simulink model "shock_absorb"  (R2020b)
settings: Solver=VariableStepAuto  StartTime=0.0  StopTime=100  RelTol=1e-3
model workspace (MAT data in the model file):
  b = Simulink.Parameter
  b.Value = 8
  b.DataType = 'auto'
  b.Dimensions = [1 1]
  k1 = Simulink.Parameter
  k1.Value = 5.71
  k1.DataType = 'auto'
  k1.Dimensions = [1 1]
  k2 = Simulink.Parameter
  k2.Value = 0.15
  k2.DataType = 'auto'
  k2.Dimensions = [1 1]
  m1 = Simulink.Parameter
  m1.Value = 330
  m1.DataType = 'auto'
  m1.Dimensions = [1 1]
  m2 = Simulink.Parameter
  m2.Value = 165
  m2.DataType = 'auto'
  m2.Dimensions = [1 1]
settings Model: Creator=shivanshu shukla  LastModifiedBy=shivanshu shukla

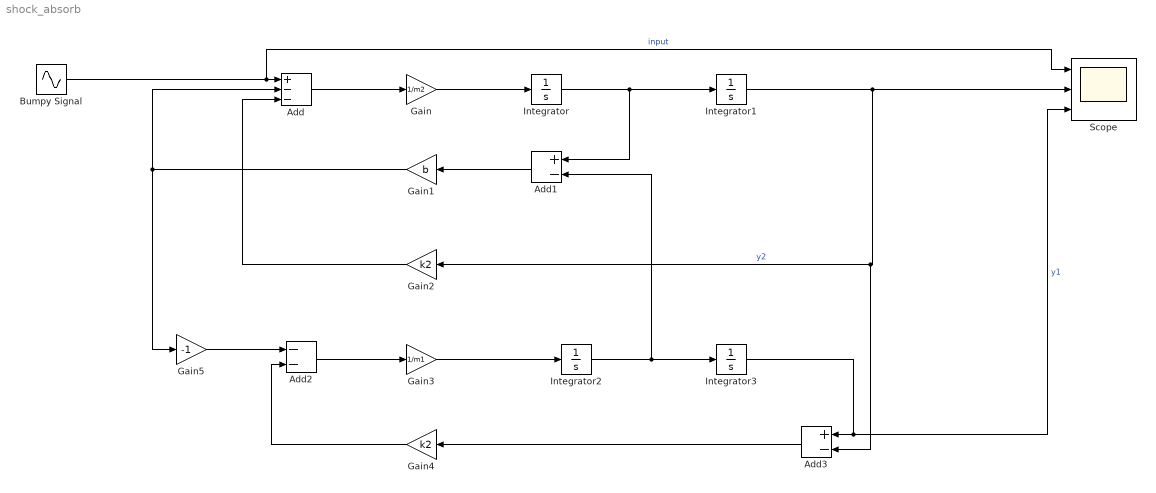
== system shock_absorb ==
  Add : Sum  Inputs=+--
  Add1 : Sum  Inputs=+-
  Add2 : Sum  Inputs=--
  Add3 : Sum  Inputs=+-
  Bumpy Signal : Sin  SampleTime=0
  Gain : Gain  Gain=1/m2
  Gain1 : Gain  Gain=b
  Gain2 : Gain  Gain=k2
  Gain3 : Gain  Gain=1/m1
  Gain4 : Gain  Gain=k2
  Gain5 : Gain  Gain=-1
  Integrator{,1..3} (4 alike) : Integrator
  Scope : Scope  NumInputPorts=3
  wires:
  Add/1 -> Gain/1
  Gain/1 -> Integrator/1
  Integrator/1 -> Add1/1, Integrator1/1
  Integrator1/1 -> Scope/2, Gain2/1, Add3/2  "y2"
  Gain1/1 -> Gain5/1, Add/2
  Add1/1 -> Gain1/1
  Gain2/1 -> Add/3
  Gain3/1 -> Integrator2/1
  Integrator2/1 -> Add1/2, Integrator3/1
  Gain5/1 -> Add2/1
  Add2/1 -> Gain3/1
  Integrator3/1 -> Scope/3, Add3/1  "y1"
  Add3/1 -> Gain4/1
  Gain4/1 -> Add2/2
  Bumpy Signal/1 -> Scope/1, Add/1  "input"
